simulink model "ncmexample"  (Simulink 7.4)
settings: Solver=ode3  StartTime=0.0  StopTime=10.0  FixedStep=0.125  RelTol=1e-3
libraries: truetime x7, NCM x1
settings Model: Creator=sf  LastModifiedBy=anton  ExtModeAutoUpdateStatusClock=off
settings OptimizationCC: InitFltsAndDblsToZero=on
settings DebuggingCC: SaveWithParameterizedLinksMsg=none
settings GRTTargetCC: TargetFcnLib=ansi_tfl_tmw.mat

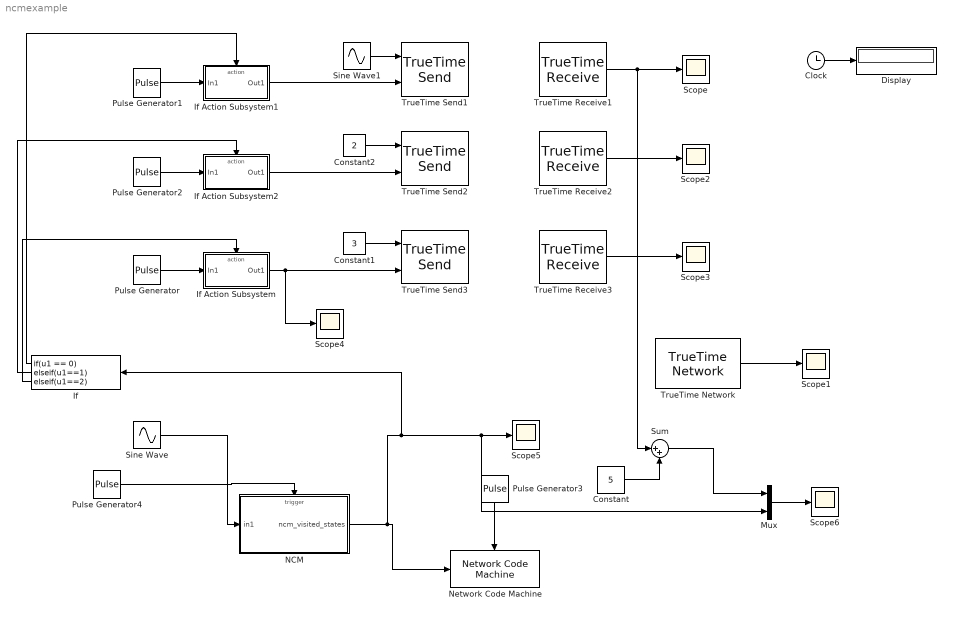
== system ncmexample ==
  Clock : Clock
      settings: Decimation=10
  Constant : Constant  Value=5  OutDataType=fixdt(1, 16)  OutScaling=2^0
  Constant1 : Constant  Value=3
  Constant2 : Constant  Value=2
  Display : Display
  If : If  IfExpression=u1 == 0  ElseIfExpressions=u1==1,u1==2  ShowElse=off
  If Action Subsystem : Subsystem  TreatAsAtomicUnit=on
  If Action Subsystem1 : Subsystem  TreatAsAtomicUnit=on
  If Action Subsystem2 : Subsystem  TreatAsAtomicUnit=on
  Mux : Mux  Inputs=2
  NCM : Stateflow chart  TreatAsAtomicUnit=on
  Network Code Machine : NCM/Network Code Machine  SystemSampleTime=-1
  Pulse Generator : DiscretePulseGenerator  PulseType=Time based  Amplitude=1  Period=0.5  PulseWidth=50  PhaseDelay=0  SampleTime=1
  Pulse Generator1 : DiscretePulseGenerator  PulseType=Time based  Amplitude=1  Period=0.5  PulseWidth=50  PhaseDelay=0  SampleTime=1
  Pulse Generator2 : DiscretePulseGenerator  PulseType=Time based  Amplitude=1  Period=0.5  PulseWidth=50  PhaseDelay=0  SampleTime=1
  Pulse Generator3 : DiscretePulseGenerator  PulseType=Time based  Amplitude=1  Period=0.25  PulseWidth=50  PhaseDelay=.5  SampleTime=1
  Pulse Generator4 : DiscretePulseGenerator  PulseType=Time based  Amplitude=1  Period=0.25  PulseWidth=50  PhaseDelay=0  SampleTime=1
  Scope{,1..6} (7 alike) : Scope
      Scope settings: YMin=0  YMax=3
      Scope2 settings: SaveName=ScopeData2
      Scope3 settings: SaveName=ScopeData3
      Scope4 settings: SaveName=ScopeData4
      Scope5 settings: SaveName=ScopeData5
      Scope6 settings: YMin=0  YMax=3  SaveName=ScopeData6
  Sine Wave : Sin  Amplitude=1  Bias=0  Frequency=1  Phase=0  Samples=10  SampleTime=0  Offset=0
  Sine Wave1 : Sin  Amplitude=1  Bias=0  Frequency=1  Phase=0  Samples=10  SampleTime=0  Offset=0
  Sum : Sum  Inputs=|++  OutDataType=fixdt(1, 16)  OutScaling=2^0
  TrueTime Network : truetime/TrueTime Network  SystemSampleTime=-1  nwtype=NCM  nwnbr=1  nnodes=3  rate=10000000  minsize=512  lossprob=0  seed=0  bandwidths=[0.5 0.5]  slotsize=512  schedule=[1 1 2]  memsize=80000  buftype=Common buffer  overflow=Retransmit  dynSchedule=0  miniSlotSize=0  NIT=0  QSortMode=FIFO  sync=0  irtSchedule=0  nrtLength=0  nodeGraph=0  scheduleoutput=on
  TrueTime Receive1 : truetime/TrueTime Receive  SystemSampleTime=-1  nwnbr=1  receiver=1  outdim=1  triggeroutput=off  senderoutput=off  lengthoutput=off  priorityoutput=off  timestampoutput=off  signalpoweroutput=off  msgIDoutput=off
  TrueTime Receive2 : truetime/TrueTime Receive  SystemSampleTime=-1  nwnbr=1  receiver=2  outdim=1  triggeroutput=off  senderoutput=off  lengthoutput=off  priorityoutput=off  timestampoutput=off  signalpoweroutput=off  msgIDoutput=off
  TrueTime Receive3 : truetime/TrueTime Receive  SystemSampleTime=-1  nwnbr=1  receiver=3  outdim=1  triggeroutput=off  senderoutput=off  lengthoutput=off  priorityoutput=off  timestampoutput=off  signalpoweroutput=off  msgIDoutput=off
  TrueTime Send1 : truetime/TrueTime Send  SystemSampleTime=-1  trigger=falling  nwnbr=1  sender=1  indim=1  recsource=internal  receiver=1  lengthsource=internal  length=1000  priosource=internal  prio=1  msgIDsource=internal  msgID=0  dynamicSegment=dynamic
  TrueTime Send2 : truetime/TrueTime Send  SystemSampleTime=-1  trigger=falling  nwnbr=1  sender=2  indim=1  recsource=internal  receiver=1  lengthsource=internal  length=1000  priosource=internal  prio=1  msgIDsource=internal  msgID=0  dynamicSegment=dynamic
  TrueTime Send3 : truetime/TrueTime Send  SystemSampleTime=-1  trigger=falling  nwnbr=1  sender=3  indim=1  recsource=internal  receiver=1  lengthsource=internal  length=1000  priosource=internal  prio=1  msgIDsource=internal  msgID=0  dynamicSegment=dynamic
  wires:
  Clock/1 -> Display/1
  TrueTime Network/1 -> Scope1/1
  Pulse Generator3/1 -> Network Code Machine/Trigger
  Sine Wave1/1 -> TrueTime Send1/1
  Constant1/1 -> TrueTime Send3/1
  Constant2/1 -> TrueTime Send2/1
  If/3 -> If Action Subsystem/Action
  If Action Subsystem/1(Out1) -> TrueTime Send3/2, Scope4/1
  If Action Subsystem2/1(Out1) -> TrueTime Send2/2
  If/2 -> If Action Subsystem2/Action
  If/1 -> If Action Subsystem1/Action
  If Action Subsystem1/1(Out1) -> TrueTime Send1/2
  Pulse Generator/1 -> If Action Subsystem/1(In1)
  Pulse Generator2/1 -> If Action Subsystem2/1(In1)
  Pulse Generator1/1 -> If Action Subsystem1/1(In1)
  TrueTime Receive1/1 -> Scope/1, Sum/1
  TrueTime Receive2/1 -> Scope2/1
  TrueTime Receive3/1 -> Scope3/1
  Pulse Generator4/1 -> NCM/Trigger
  NCM/1(ncm_visited_states) -> Network Code Machine/1, If/1, Scope5/1, Mux/2
  Sine Wave/1 -> NCM/1(in1)
  Mux/1 -> Scope6/1
  Constant/1 -> Sum/2
  Sum/1 -> Mux/1

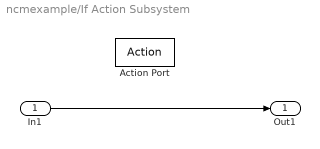
== system ncmexample/If Action Subsystem ==
  In1 : Inport  OutDataType=fixdt(1, 16)  OutScaling=2^0
  Action Port : ActionPort  ActionType=elseif
  Out1 : Outport  OutDataType=fixdt(1, 16)  OutScaling=2^0
  wires:
  In1/1 -> Out1/1

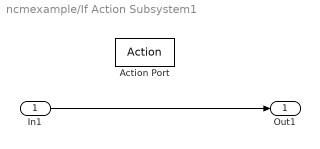
== system ncmexample/If Action Subsystem1 ==
  In1 : Inport  OutDataType=fixdt(1, 16)  OutScaling=2^0
  Action Port : ActionPort  ActionType=then
  Out1 : Outport  OutDataType=fixdt(1, 16)  OutScaling=2^0
  wires:
  In1/1 -> Out1/1

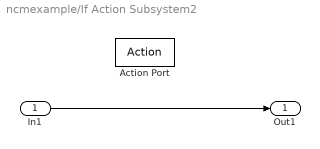
== system ncmexample/If Action Subsystem2 ==
  In1 : Inport  OutDataType=fixdt(1, 16)  OutScaling=2^0
  Action Port : ActionPort  ActionType=elseif
  Out1 : Outport  OutDataType=fixdt(1, 16)  OutScaling=2^0
  wires:
  In1/1 -> Out1/1

== stateflow chart NCM ==
  state NCM
    state node3
      entry:
      ncm_visited_states=2;
    state node2
      entry: ncm_visited_states= 1;
    state node1
      entry: ncm_visited_states=0;
    state saved_state
      entry: ncm_visited_states=0;
    node3 -> node1 : after(1,CLOCK)...
    (default) -> node1
    node1 -> node2 : after(1,CLOCK)...
    node2 -> node3 [order 1] : after(1,CLOCK)...
        | [in1 > .5]
    node2 -> saved_state [order 2] : after(1,CLOCK)...
        | [ in1 <= .5]
    saved_state -> node1
  data: ncm_visited_states output double; in1 input double
  events: CLOCK input FALLING_EDGE_EVENT
